simulink model "MAVDynamics_2"  (R2017b)
settings: Solver=ode4  StartTime=0.0  StopTime=20  FixedStep=sim_step  RelTol=1e-3  EnableMultiTasking=on
undefined symbols (not defined in the file): g, J, m
settings Model: Creator=Burak  LastModifiedBy=buyue
settings DataIOCC: LimitDataPoints=on  SaveFormat=Array
settings OptimizationCC: LifeSpan=inf
settings DebuggingCC: UnderspecifiedInitializationDetection=Classic  MergeDetectMultiDrivingBlocksExec=none  SolverPrmCheckMsg=warning  StateNameClashWarn=warning  SFUnexpectedBacktrackingDiag=warning  SFNoUnconditionalDefaultTransitionDiag=warning  SFExecutionAtInitializationDiag=none
settings HardwareCC: ProdBitPerPointer=32  ProdBitPerSizeT=32  ProdBitPerPtrDiffT=32  ProdLargestAtomicFloat=None  ProdIntDivRoundTo=Undefined  ProdEndianess=Unspecified  ProdWordSize=32  ProdHWDeviceType=32-bit Generic
settings ModelReferenceCC: PropagateSignalLabelsOutOfModel=off
settings CodeAppCC: StateflowObjectComments=on
settings GRTTargetCC: TargetLangStandard=C89/C90 (ANSI)  GeneratePreprocessorConditionals=Disable all
settings ConfigComp: CovMetricSettings=dw  CovHtmlReporting=on  CovSaveCumulativeToWorkspaceVar=on  CovSaveSingleToWorkspaceVar=on  CovExternalEMLEnable=off

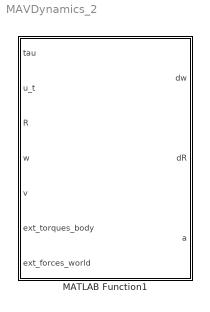
== system MAVDynamics_2 ==
  MATLAB Function1 : MATLAB Function  Description=|  TreatAsAtomicUnit=on
      | % Dynamics of a MAV-VTOL.
      | % Body is subject to one thrust and three torques, hence four control
      | % inputs
      | % In this course, these four inputs are resulting effect of spinning
      | % propellers. For a quadrotor, there are four of them. It could be a
      | % hexarotor, octorotor, etc. As long as the propellers are placed in a
      | % collinear way, following dynamics holds.
      | % Code part of Lecture IAR @IST-Uni Stuttgart
      | % Author: Burak Yueksel

== matlab function MAVDynamics_2/MATLAB Function1 ==
  data: tau input; dw output; u_t input; R input; w input; v input; ext_torques_body input; ext_forces_world input; m parameter; J parameter; g parameter; dR output; a output
function [dw, dR, a] = MAVDynamics(tau,u_t,R,w,v,ext_torques_body,ext_forces_world,m,J,g)
% Dynamics of a MAV-VTOL.
% Body is subject to one thrust and three torques, hence four control
% inputs
% In this course, these four inputs are resulting effect of spinning
% propellers. For a quadrotor, there are four of them. It could be a
% hexarotor, octorotor, etc. As long as the propellers are placed in a
% collinear way, following dynamics holds.
% Code part of Lecture IAR @IST-Uni Stuttgart
% Author: Burak Yueksel
u_t = -u_t; % comment this out if NH is commenting positive thrust
a = g*[0;0;1]-u_t/m*R*[0;0;1] + ext_forces_world/m;
Sw = [0     -w(3)   w(2);
      w(3)   0     -w(1);
     -w(2)  w(1)      0];
% init integrator of R with eye(3)
dR = R*Sw;
dw = inv(J)*(-Sw*J*w+tau + ext_torques_body);
